simulink model "galvoMdl"  (R2015a)
settings: Solver=ode45  StartTime=0.0  StopTime=10.0  RelTol=1e-3
undefined symbols (not defined in the file): BF, JR, KEL, KEMF, KFR, KME, KPD, KTB, L, RL
settings Model: Creator=mainster  LastModifiedBy=mainster
settings DebuggingCC: UnderspecifiedInitializationDetection=Classic  MergeDetectMultiDrivingBlocksExec=none  SolverPrmCheckMsg=warning  StateNameClashWarn=warning

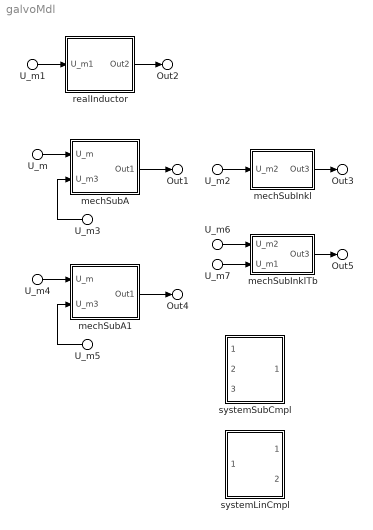
== system galvoMdl ==
  U_m : Inport
  U_m2 : Inport  Port=2
  U_m3 : Inport  Port=3
  U_m1 : Inport  Port=4
  U_m4 : Inport  Port=5
  U_m5 : Inport  Port=6
  U_m6 : Inport  Port=7
  U_m7 : Inport  Port=8
  mechSubA : Subsystem
  mechSubA1 : Subsystem
  mechSubInkl : Subsystem
  mechSubInklTb : Subsystem
  realInductor : Subsystem
      settings: AttributesFormatString=%<BlockType>
  systemLinCmpl : Subsystem
  systemSubCmpl : Subsystem
  Out1 : Outport
  Out3 : Outport  Port=2
  Out2 : Outport  Port=3
  Out4 : Outport  Port=4
  Out5 : Outport  Port=5
  wires:
  U_m1/1 -> realInductor/1(U_m1)
  realInductor/1(Out2) -> Out2/1
  U_m2/1 -> mechSubInkl/1(U_m2)
  mechSubInkl/1(Out3) -> Out3/1
  U_m/1 -> mechSubA/1(U_m)
  U_m3/1 -> mechSubA/2(U_m3)
  mechSubA/1(Out1) -> Out1/1
  U_m4/1 -> mechSubA1/1(U_m)
  U_m5/1 -> mechSubA1/2(U_m3)
  mechSubA1/1(Out1) -> Out4/1
  U_m6/1 -> mechSubInklTb/1(U_m2)
  mechSubInklTb/1(Out3) -> Out5/1
  U_m7/1 -> mechSubInklTb/2(U_m1)

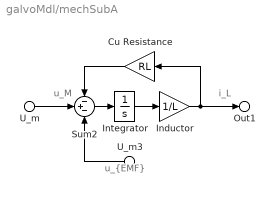
== system galvoMdl/mechSubA ==
  note: u_M
  note: i_L
  note: u_{EMF}
  U_m : Inport
  U_m3 : Inport  Port=2
  Cu Resistance : Gain  Gain=RL
  Inductor : Gain  Gain=1/L
  Integrator : Integrator
  Sum2 : Sum  Inputs=-+-
  Out1 : Outport
  wires:
  Sum2/1 -> Integrator/1
  Cu Resistance/1 -> Sum2/1
  Integrator/1 -> Inductor/1
  U_m3/1 -> Sum2/3
  U_m/1 -> Sum2/2
  Inductor/1 -> Out1/1, Cu Resistance/1

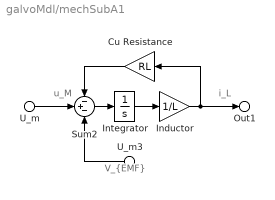
== system galvoMdl/mechSubA1 ==
  note: u_M
  note: i_L
  note: V_{EMF}
  U_m : Inport
  U_m3 : Inport  Port=2
  Cu Resistance : Gain  Gain=RL
  Inductor : Gain  Gain=1/L
  Integrator : Integrator
  Sum2 : Sum  Inputs=-+-
  Out1 : Outport
  wires:
  Sum2/1 -> Integrator/1
  Cu Resistance/1 -> Sum2/1
  Integrator/1 -> Inductor/1
  U_m3/1 -> Sum2/3
  U_m/1 -> Sum2/2
  Inductor/1 -> Out1/1, Cu Resistance/1

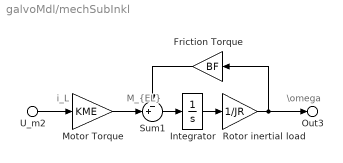
== system galvoMdl/mechSubInkl ==
  note: M_{EL}
  note: \omega
  note: i_L
  U_m2 : Inport
  Friction Torque : Gain  Gain=BF
  Integrator : Integrator
  Motor Torque : Gain  Gain=KME
  Rotor inertial load : Gain  Gain=1/JR
  Sum1 : Sum  Inputs=-+|
  Out3 : Outport
  wires:
  Sum1/1 -> Integrator/1
  Integrator/1 -> Rotor inertial load/1
  Friction Torque/1 -> Sum1/1
  U_m2/1 -> Motor Torque/1
  Motor Torque/1 -> Sum1/2
  Rotor inertial load/1 -> Out3/1, Friction Torque/1

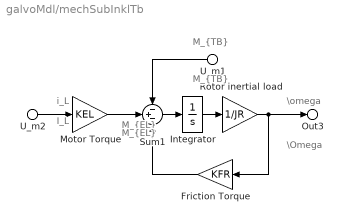
== system galvoMdl/mechSubInklTb ==
  note: M_{EL}
  note: \omega
  note: i_L
  note: I_L
  note: M_{EL}
  note: \Omega
  note: M_{TB}
  note: M_{TB}
  U_m2 : Inport
  U_m1 : Inport  Port=2
  Friction Torque : Gain  Gain=KFR
  Integrator : Integrator
  Motor Torque : Gain  Gain=KEL
  Rotor inertial load : Gain  Gain=1/JR
  Sum1 : Sum  Inputs=-+-
  Out3 : Outport
  wires:
  Sum1/1 -> Integrator/1
  Integrator/1 -> Rotor inertial load/1
  Friction Torque/1 -> Sum1/3
  U_m2/1 -> Motor Torque/1
  Motor Torque/1 -> Sum1/2
  Rotor inertial load/1 -> Out3/1, Friction Torque/1
  U_m1/1 -> Sum1/1

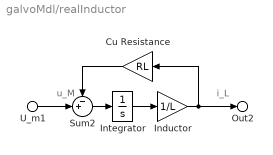
== system galvoMdl/realInductor ==
  note: u_M
  note: i_L
  U_m1 : Inport
  Cu Resistance : Gain  Gain=RL
  Inductor : Gain  Gain=1/L
  Integrator : Integrator
  Sum2 : Sum  Inputs=-+|
  Out2 : Outport
  wires:
  U_m1/1 -> Sum2/2
  Sum2/1 -> Integrator/1
  Inductor/1 -> Out2/1, Cu Resistance/1
  Integrator/1 -> Inductor/1
  Cu Resistance/1 -> Sum2/1

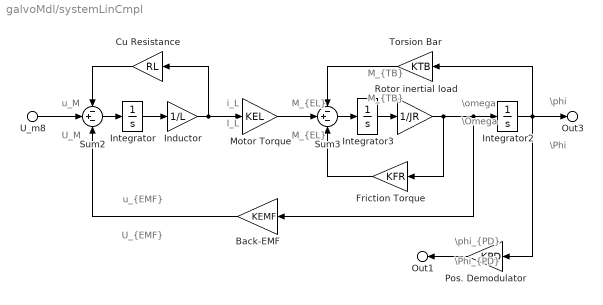
== system galvoMdl/systemLinCmpl ==
  note: \Phi
  note: \phi
  note: u_M
  note: M_{EL}
  note: \omega
  note: i_L
  note: I_L
  note: M_{EL}
  note: \Omega
  note: M_{TB}
  note: M_{TB}
  note: U_M
  note: u_{EMF}
  note: U_{EMF}
  note: \Phi_{PD}
  note: \phi_{PD}
  U_m8 : Inport
  Back-EMF : Gain  Gain=KEMF
  Cu Resistance : Gain  Gain=RL
  Friction Torque : Gain  Gain=KFR
  Inductor : Gain  Gain=1/L
  Integrator : Integrator
  Integrator2 : Integrator
  Integrator3 : Integrator
  Motor Torque : Gain  Gain=KEL
  Pos. Demodulator : Gain  Gain=KPD
  Rotor inertial load : Gain  Gain=1/JR
  Sum2 : Sum  Inputs=-+-
  Sum3 : Sum  Inputs=-+-
  Torsion Bar : Gain  Gain=KTB
  Out3 : Outport
  Out1 : Outport  Port=2
  wires:
  Back-EMF/1 -> Sum2/3
  Sum2/1 -> Integrator/1
  Cu Resistance/1 -> Sum2/1
  U_m8/1 -> Sum2/2
  Integrator/1 -> Inductor/1
  Inductor/1 -> Motor Torque/1, Cu Resistance/1
  Motor Torque/1 -> Sum3/2
  Integrator2/1 -> Pos. Demodulator/1, Torsion Bar/1, Out3/1
  Sum3/1 -> Integrator3/1
  Integrator3/1 -> Rotor inertial load/1
  Friction Torque/1 -> Sum3/3
  Torsion Bar/1 -> Sum3/1
  Rotor inertial load/1 -> Back-EMF/1, Integrator2/1, Friction Torque/1
  Pos. Demodulator/1 -> Out1/1

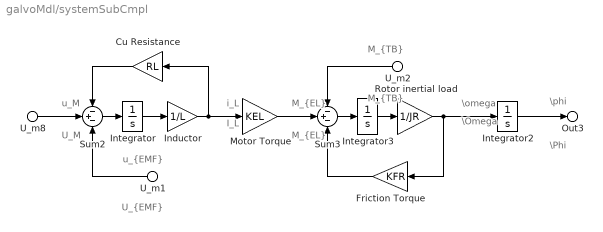
== system galvoMdl/systemSubCmpl ==
  note: \Phi
  note: \phi
  note: u_M
  note: u_{EMF}
  note: M_{EL}
  note: \omega
  note: i_L
  note: I_L
  note: M_{EL}
  note: \Omega
  note: M_{TB}
  note: M_{TB}
  note: U_M
  note: U_{EMF}
  U_m8 : Inport
  U_m1 : Inport  Port=2
  U_m2 : Inport  Port=3
  Cu Resistance : Gain  Gain=RL
  Friction Torque : Gain  Gain=KFR
  Inductor : Gain  Gain=1/L
  Integrator : Integrator
  Integrator2 : Integrator
  Integrator3 : Integrator
  Motor Torque : Gain  Gain=KEL
  Rotor inertial load : Gain  Gain=1/JR
  Sum2 : Sum  Inputs=-+-
  Sum3 : Sum  Inputs=-+-
  Out3 : Outport
  wires:
  U_m1/1 -> Sum2/3
  Sum2/1 -> Integrator/1
  Cu Resistance/1 -> Sum2/1
  U_m8/1 -> Sum2/2
  Integrator/1 -> Inductor/1
  Inductor/1 -> Motor Torque/1, Cu Resistance/1
  Motor Torque/1 -> Sum3/2
  Integrator2/1 -> Out3/1
  Sum3/1 -> Integrator3/1
  Integrator3/1 -> Rotor inertial load/1
  Friction Torque/1 -> Sum3/3
  U_m2/1 -> Sum3/1
  Rotor inertial load/1 -> Integrator2/1, Friction Torque/1
